simulink model "v1"  (R2024a)
settings: Solver=VariableStepAuto  StartTime=0.0  StopTime=10  RelTol=1e-3
model workspace (MAT data in the model file):
  Kd_val1 = 5
  Kd_val2 = 5
  Ki_val1 = 5
  Ki_val2 = 5
  Kp_val1 = 400
  Kp_val2 = 500
settings Model: Creator=HP  LastModifiedBy=HP

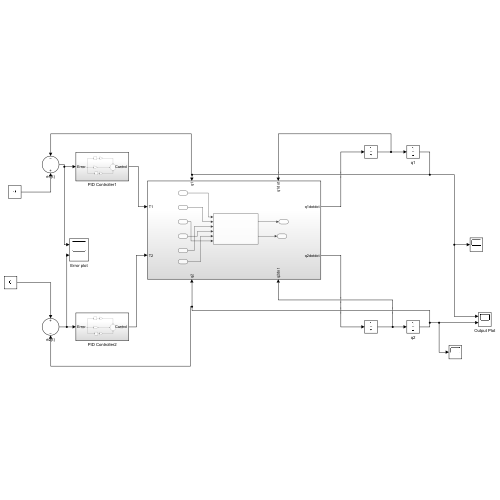
[thumbnail: Simulink's stored preview of the top-level diagram]
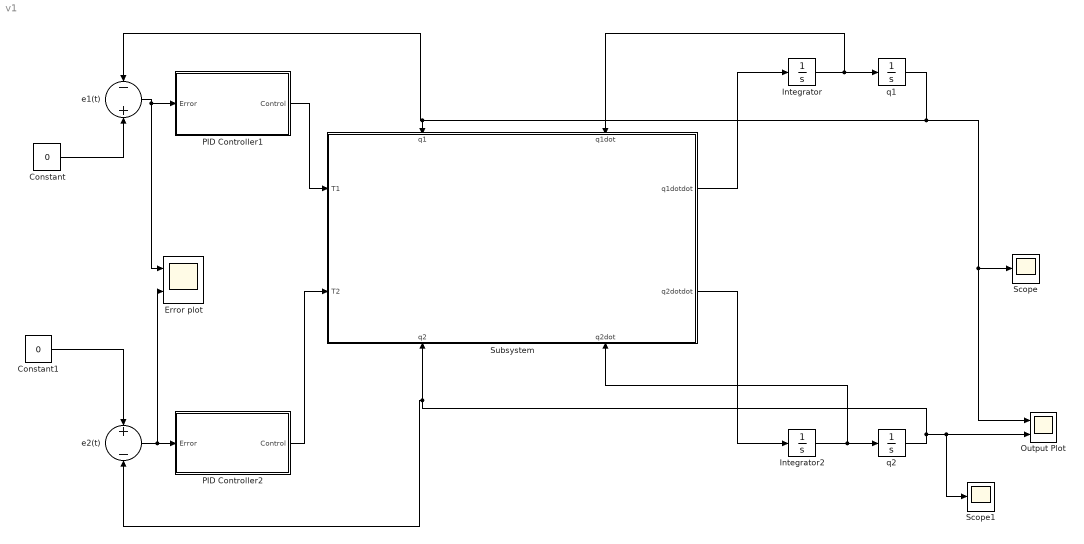
== system v1 ==
  Constant : Constant  Value=0
  Constant1 : Constant  Value=0
  Error plot : Scope  NumInputPorts=2
  Integrator : Integrator
  Integrator2 : Integrator
  Output Plot : Scope  NumInputPorts=2
  PID Controller1 : Subsystem
  PID Controller2 : Subsystem
  Scope : Scope
  Scope1 : Scope
  Subsystem : Subsystem
      settings: PortSchema="{\"entries\":[{\"content\":{\"sides\":[{\"content\":{\"connectorIds\":[\"In1\",\"In2\"]},\"type\":\"ConnectorPlacement.EquallySpacedRectSide\",\"uuid\":\"83594621-0f92-4348-9a89-2feac7dea3e4\"},{\"content\":{\"connectorIds\":[\"Out1\",\"Out2\"],\"side\":\"RIGHT\"},\"type\":\"ConnectorPlacement.EquallySpacedRectSide\",\"uuid\":\"4de7f8ec-c0f8-4805-ba7c-b4184f5c99cc\"},{\"content\":{\"connectorIds\":[\"In3\",\"In4\"],\"side\":\"TOP\"},\"type\":\"ConnectorPlacement.EquallySpacedRectSide\",\"uuid\":\"f1cccd6e-0645-4752-b4d0-b5009957b0cd\"},{\"content\":{\"connectorIds\":[\"In5\",\"In6\"],\"side\":\"BOTTOM\"},\"type\":\"ConnectorPlacement.EquallySpacedRectSide\",\"uuid\":\"5fe903eb-3ecc-42a3-872d-334923a10ab8\"}]},\"type\":\"ConnectorPlacement.EquallySpacedConnector\",\"uuid\":\"79d4f09b-c46e-4514-82d4-34ce1142f6aa\"}],\"packageUris\":[\"http://schema.mathworks.com/mf0/Connector/R2020b\"],\"version\":\"1.0\"}"
  e1(t) : Sum  Inputs=-+
  e2(t) : Sum  Inputs=+-
  q1 : Integrator  InitialCondition=0.1
  q2 : Integrator  InitialCondition=0.1
  wires:
  e1(t)/1 -> Error plot/1, PID Controller1/1(Error)
  PID Controller2/1(Control) -> Subsystem/2(T2)
  PID Controller1/1(Control) -> Subsystem/1(T1)
  Subsystem/2(q2dotdot) -> Integrator2/1
  Subsystem/1(q1dotdot) -> Integrator/1
  Integrator2/1 -> Subsystem/6(q2dot), q2/1
  Integrator/1 -> Subsystem/4(q1dot), q1/1
  q1/1 -> Scope/1, Output Plot/1, e1(t)/1, Subsystem/3(q1)
  q2/1 -> e2(t)/2, Subsystem/5(q2), Scope1/1, Output Plot/2
  Constant/1 -> e1(t)/2
  Constant1/1 -> e2(t)/1
  e2(t)/1 -> Error plot/2, PID Controller2/1(Error)

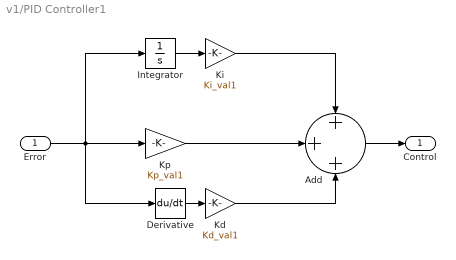
== system v1/PID Controller1 ==
  Error : Inport
  Add : Sum  Inputs=+++
  Derivative : Derivative
  Integrator : Integrator
  Kd : Gain  Gain=Kd_val1
  Ki : Gain  Gain=Ki_val1
  Kp : Gain  Gain=Kp_val1
  Control : Outport
  wires:
  Error/1 -> Kp/1, Derivative/1, Integrator/1
  Integrator/1 -> Ki/1
  Derivative/1 -> Kd/1
  Kd/1 -> Add/3
  Kp/1 -> Add/2
  Ki/1 -> Add/1
  Add/1 -> Control/1

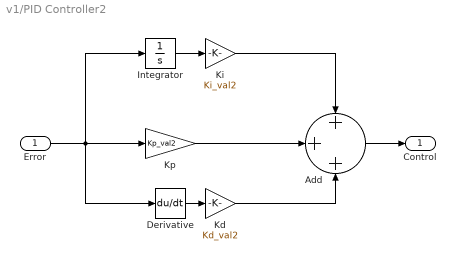
== system v1/PID Controller2 ==
  Error : Inport
  Add : Sum  Inputs=+++
  Derivative : Derivative
  Integrator : Integrator
  Kd : Gain  Gain=Kd_val2
  Ki : Gain  Gain=Ki_val2
  Kp : Gain  Gain=Kp_val2
  Control : Outport
  wires:
  Error/1 -> Kp/1, Derivative/1, Integrator/1
  Integrator/1 -> Ki/1
  Derivative/1 -> Kd/1
  Kd/1 -> Add/3
  Kp/1 -> Add/2
  Ki/1 -> Add/1
  Add/1 -> Control/1

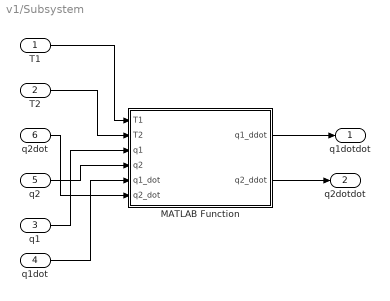
== system v1/Subsystem ==
  T1 : Inport
  T2 : Inport  Port=2
  q1 : Inport  Port=3
  q1dot : Inport  Port=4
  q2 : Inport  Port=5
  q2dot : Inport  Port=6
  MATLAB Function : MATLAB Function  TreatAsAtomicUnit=on
  q1dotdot : Outport
  q2dotdot : Outport  Port=2
  wires:
  T2/1 -> MATLAB Function/2(T2)
  T1/1 -> MATLAB Function/1(T1)
  q1dot/1 -> MATLAB Function/5(q1_dot)
  q1/1 -> MATLAB Function/3(q1)
  q2/1 -> MATLAB Function/4(q2)
  q2dot/1 -> MATLAB Function/6(q2_dot)
  MATLAB Function/1(q1_ddot) -> q1dotdot/1
  MATLAB Function/2(q2_ddot) -> q2dotdot/1

== matlab function v1/Subsystem/MATLAB Function ==
  data: T1 input; q1_ddot output; T2 input; q1 input; q2 input; q1_dot input; q2_dot input; q2_ddot output
function [q1_ddot, q2_ddot] = compute_acceleration(T1, T2, q1, q2, q1_dot, q2_dot)
    % Define constants
    m1 = 10; % kg
    m2 = 5;  % kg
    l1 = 0.2; % m
    l2 = 0.1; % m
    g = 9.81; % m/s^2
    
    % Inertia matrix M
    M11 = (m1 + m2)*l1^2 + m2*l2*(l2 + 2*l1*cos(q2));
    M12 = m2*l2*(l2 + l1*cos(q2));
    M22 = m2*l2^2;
    
    M = [M11 M12; M12 M22];
    
    % Coriolis and Centrifugal matrix C
    C11 = -m2*l1*l2*sin(q2)*q2_dot;
    C12 = -m2*l1*l2*sin(q2)*(q1_dot + q2_dot);
    C21 = 0;
    C22 = m2*l1*l2*sin(q2)*q1_dot;
    
    C = [C11 C12; C21 C22];
    
    % Gravity vector G
    G1 = m1*l1*g*cos(q1) + m2*g*(l2*cos(q1 + q2) + l1*cos(q1));
    G2 = m2*g*l2*cos(q1 + q2);
    
    G = [G1; G2];
    
    % Torque input vector
    tau = [T1; T2];
    
    % Joint velocities
    q_dot = [q1_dot; q2_dot];
    
    % Compute q_ddot using the equation
    q_ddot = (tau - (C*q_dot + G))./M;
    
    % Separate outputs for q1_ddot and q2_ddot
    q1_ddot = q_ddot(1);
    q2_ddot = q_ddot(2);
end
